simulink subsystem "MultibodySuspensionSSC"  (R2023b)
settings: Solver=VariableStepAuto  StartTime=0.0  StopTime=10.0  RelTol=1e-3
undefined symbols (not defined in the file): EnvGrvty, FrntRef, LAc, LAf, LAr, PlntVehDstCGFrntAxl, PlntVehDstCGRearAxl, PlntVehMass, PlntVehMultiBody, PlntVehMultiBodyGeom, RearRef, StrRodFL, StrRodFR, StrRodRL, StrRodRR, UAc, UAf, UAr, WheelFL, WheelFR, WheelRL, WheelRR, X, Y, Z
libraries: sm_lib x450, fl_lib x96, nesl_utility x64, sdl_lib x8
(part 1 of 18)
settings Model: Creator=The MathWorks, Inc.  LastModifiedBy=The MathWorks, Inc.
settings OptimizationCC: ReuseModelBlockBuffer=off
settings DebuggingCC: SubsystemReferenceDiagnosticForUnitTest=warning

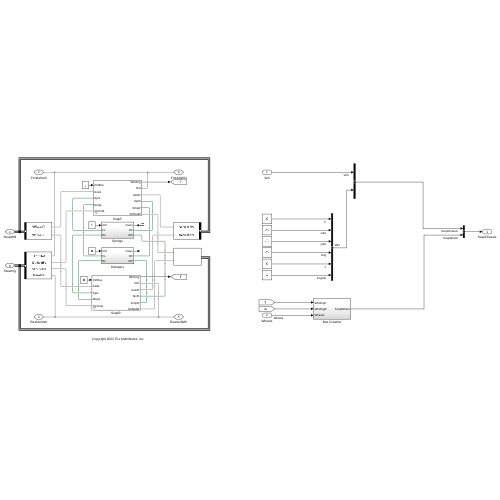
[thumbnail: Simulink's stored preview of the top-level diagram]
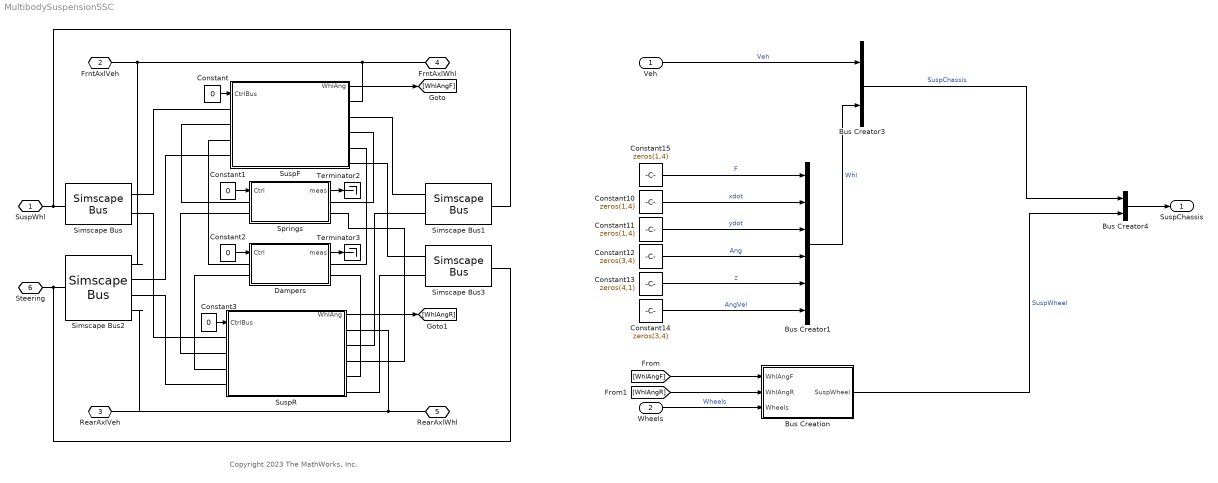
== system MultibodySuspensionSSC ==
  note: Copyright 2023 The MathWorks, Inc.
  Veh : Inport
  Wheels : Inport  Port=2
  Bus Creator1 : BusCreator  Inputs=6
  Bus Creator3 : BusCreator  Inputs=2
  Bus Creator4 : BusCreator  Inputs=2
  Bus Creation : Subsystem
  Constant{,1..3} (4 alike) : Constant  Value=0  SampleTime=-1
  Constant10 : Constant  Value=zeros(1,4)  SampleTime=-1
  Constant11 : Constant  Value=zeros(1,4)  SampleTime=-1
  Constant12 : Constant  Value=zeros(3,4)  SampleTime=-1
  Constant13 : Constant  Value=zeros(4,1)  SampleTime=-1
  Constant14 : Constant  Value=zeros(3,4)  SampleTime=-1
  Constant15 : Constant  Value=zeros(1,4)  SampleTime=-1
  Dampers : Subsystem
  Simscape Bus : SimscapeBus  HierarchyStrings=WheelFL;WheelRL
  Simscape Bus1 : SimscapeBus  HierarchyStrings=WheelFR;WheelRR
  Simscape Bus2 : SimscapeBus  HierarchyStrings=FrntRef;StrRodFL;StrRodRL;RearRef
  Simscape Bus3 : SimscapeBus  HierarchyStrings=StrRodFR;StrRodRR
  Springs : Subsystem
  SuspF : Subsystem  mask(Suspension and Steering){Susp=PlntVehMultiBody.Chassis.SuspF, Init=[0 0 0], InitTriggerDropdown=1}
      mask prompts: Susp "Suspension Parameters"; Init "Initial Values"; InitTriggerDropdown "Initialization Trigger Dropdown"
      mask help: Suspension and steering system for front or rear axle.
      mask init:
      | % curblk = gcb;
      | % Trigger Mask Initialization for 
      | % variant subsystems below this level
      | % sm_car_4post_lib_maskInitTrigger(curblk)
      settings: LibrarySourceBlock=sm_car_4post_lib/Suspension and Steering
      mask TypeOptions InitTriggerDropdown: 0 | 1
  SuspR : Subsystem  mask(Suspension and Steering){Susp=PlntVehMultiBody.Chassis.SuspR, Init=[0 0 0], InitTriggerDropdown=1}
      mask prompts: Susp "Suspension Parameters"; Init "Initial Values"; InitTriggerDropdown "Initialization Trigger Dropdown"
      mask help: Suspension and steering system for front or rear axle.
      mask init:
      | % curblk = gcb;
      | % Trigger Mask Initialization for 
      | % variant subsystems below this level
      | % sm_car_4post_lib_maskInitTrigger(curblk)
      settings: LibrarySourceBlock=sm_car_4post_lib/Suspension and Steering
      mask TypeOptions InitTriggerDropdown: 0 | 1
  Terminator2 : Terminator
  Terminator3 : Terminator
  SuspWhl : PMIOPort  Side=Right
  FrntAxlVeh : PMIOPort  Port=2  Side=Left
  RearAxlVeh : PMIOPort  Port=3  Side=Left
  FrntAxlWhl : PMIOPort  Port=4  Side=Right
  RearAxlWhl : PMIOPort  Port=5  Side=Right
  Steering : PMIOPort  Port=6  Side=Left
  SuspChassis : Outport
  wires:
  Constant10/1 -> Bus Creator1/2  "xdot"
  Veh/1 -> Bus Creator3/1  "Veh"
  Bus Creator3/1 -> Bus Creator4/1  "SuspChassis"
  Bus Creator4/1 -> SuspChassis/1
  Bus Creator1/1 -> Bus Creator3/2  "Whl"
  Constant11/1 -> Bus Creator1/3  "ydot"
  Constant12/1 -> Bus Creator1/4  "Ang"
  Constant13/1 -> Bus Creator1/5  "z"
  Constant14/1 -> Bus Creator1/6  "AngVel"
  Constant15/1 -> Bus Creator1/1  "F"
  Springs/1(meas) -> Terminator2/1
  Dampers/1(meas) -> Terminator3/1
  Constant1/1 -> Springs/1(Ctrl)
  Constant2/1 -> Dampers/1(Ctrl)
  Constant3/1 -> SuspR/1(CtrlBus)
  Constant/1 -> SuspF/1(CtrlBus)
  SuspF/1(WhlAng) -> [WhlAngF]
  SuspR/1(WhlAng) -> [WhlAngR]
  [WhlAngF] -> Bus Creation/1(WhlAngF)
  [WhlAngR] -> Bus Creation/2(WhlAngR)
  Wheels/1 -> Bus Creation/3(Wheels)  "Wheels"
  Bus Creation/1(SuspWheel) -> Bus Creator4/2  "SuspWheel"
  connections:
  Simscape Bus2/RConn1 -- Simscape Bus3/RConn1 -- Steering/RConn1
  SuspF/RConn1 -- FrntAxlVeh/RConn1 -- Simscape Bus2/LConn1 -- FrntAxlWhl/RConn1
  SuspR/RConn1 -- RearAxlWhl/RConn1 -- RearAxlVeh/RConn1 -- Simscape Bus2/LConn4
  SuspWhl/RConn1 -- Simscape Bus1/RConn1 -- Simscape Bus/RConn1
  SuspR/LConn4 -- Simscape Bus2/LConn3
  SuspR/RConn5 -- Simscape Bus3/LConn2
  SuspF/RConn5 -- Simscape Bus3/LConn1
  SuspF/LConn4 -- Simscape Bus2/LConn2
  Springs/LConn2 -- SuspR/LConn2
  Springs/RConn2 -- SuspR/RConn3
  SuspR/RConn4 -- Dampers/RConn2
  SuspR/LConn3 -- Dampers/LConn2
  SuspF/LConn2 -- Springs/LConn1
  SuspF/RConn3 -- Springs/RConn1
  SuspF/LConn3 -- Dampers/LConn1
  SuspF/RConn4 -- Dampers/RConn1
  SuspF/LConn1 -- Simscape Bus/LConn1
  Simscape Bus/LConn2 -- SuspR/LConn1
  SuspF/RConn2 -- Simscape Bus1/LConn1
  Simscape Bus1/LConn2 -- SuspR/RConn2

== system MultibodySuspensionSSC/Bus Creation ==
  WhlAngF : Inport
  WhlAngR : Inport  Port=2
  Wheels : Inport  Port=3
  Bus Creator : BusCreator  Inputs=8
  Bus Selector : BusSelector  OutputSignals=Wheels.Gamma
  Constant{4..9} (6 alike) : Constant  Value=zeros(1,4)  SampleTime=-1
  Convert +Z down : UnaryMinus
  Convert +Z down1 : UnaryMinus
  Matrix Concatenate : Concatenate  Mode=Multidimensional array
  Matrix Concatenate1 : Concatenate  Mode=Multidimensional array  ConcatenateDimension=2
  Reshape : Reshape  OutputDimensionality=Row vector (2-D)
  SuspWheel : Outport
  wires:
  Constant5/1 -> Bus Creator/3  "Vx"
  Wheels/1 -> Bus Selector/1, Bus Creator/8
  Bus Selector/1 -> Reshape/1  "<Gamma>"
  Constant4/1 -> Bus Creator/2  "YawRate"
  Constant8/1 -> Bus Creator/6  "Fext"
  Reshape/1 -> Matrix Concatenate/1
  Matrix Concatenate/1 -> Bus Creator/1  "WhlAng"
  Constant6/1 -> Bus Creator/4  "Vy"
  WhlAngF/1 -> Convert +Z down/1
  Constant9/1 -> Bus Creator/7  "dz"
  Constant7/1 -> Bus Creator/5  "Vz"
  Matrix Concatenate1/1 -> Matrix Concatenate/2
  Convert +Z down/1 -> Matrix Concatenate1/1
  Convert +Z down1/1 -> Matrix Concatenate1/2
  Bus Creator/1 -> SuspWheel/1  "SuspWheel"
  WhlAngR/1 -> Convert +Z down1/1

== system MultibodySuspensionSSC/Dampers ==
  Ctrl : Inport
  Independent : Subsystem  VariantControl=Independent
  Terminator : Terminator
  FL : PMIOPort  Side=Left
  FR : PMIOPort  Port=2  Side=Right
  RL : PMIOPort  Port=3  Side=Left
  RR : PMIOPort  Port=4  Side=Right
  meas : Outport  VectorParamsAs1DForOutWhenUnconnected=off
  wires:
  Ctrl/1 -> Terminator/1
  Independent/1(meas) -> meas/1
  connections:
  Independent/RConn2 -- RR/RConn1
  Independent/RConn1 -- FR/RConn1
  Independent/LConn2 -- RL/RConn1
  Independent/LConn1 -- FL/RConn1

== system MultibodySuspensionSSC/Springs ==
  Ctrl : Inport
  Independent : Subsystem  VariantControl=Independent
  Terminator : Terminator
  FL : PMIOPort  Side=Left
  FR : PMIOPort  Port=2  Side=Right
  RL : PMIOPort  Port=3  Side=Left
  RR : PMIOPort  Port=4  Side=Right
  meas : Outport  VectorParamsAs1DForOutWhenUnconnected=off
  wires:
  Ctrl/1 -> Terminator/1
  Independent/1(meas) -> meas/1
  connections:
  Independent/RConn2 -- RR/RConn1
  Independent/RConn1 -- FR/RConn1
  Independent/LConn1 -- FL/RConn1
  Independent/LConn2 -- RL/RConn1

== system MultibodySuspensionSSC/SuspF ==
  CtrlBus : Inport
  Linkage : Subsystem  VariantControl=Linkage
  Terminator : Terminator
  AxleL : PMIOPort  Side=Left
  Ref : PMIOPort  Port=2  Side=Right
  AxleR : PMIOPort  Port=3  Side=Right
  SprL : PMIOPort  Port=4  Side=Left
  SprR : PMIOPort  Port=5  Side=Right
  DmpL : PMIOPort  Port=6  Side=Left
  DmpR : PMIOPort  Port=7  Side=Right
  StrRodL : PMIOPort  Port=8  Side=Left
  StrRodR : PMIOPort  Port=9  Side=Right
  WhlAng : Outport
  wires:
  CtrlBus/1 -> Terminator/1
  Linkage/1(WhlAng) -> WhlAng/1
  connections:
  Linkage/RConn5 -- StrRodR/RConn1
  StrRodL/RConn1 -- Linkage/LConn4
  Linkage/LConn3 -- DmpL/RConn1
  Linkage/RConn2 -- AxleR/RConn1
  Linkage/LConn2 -- SprL/RConn1
  Linkage/RConn4 -- DmpR/RConn1
  Linkage/RConn3 -- SprR/RConn1
  Linkage/RConn1 -- Ref/RConn1
  Linkage/LConn1 -- AxleL/RConn1

== system MultibodySuspensionSSC/SuspR ==
  CtrlBus : Inport
  Linkage : Subsystem  VariantControl=Linkage
  Terminator : Terminator
  AxleL : PMIOPort  Side=Left
  Ref : PMIOPort  Port=2  Side=Right
  AxleR : PMIOPort  Port=3  Side=Right
  SprL : PMIOPort  Port=4  Side=Left
  SprR : PMIOPort  Port=5  Side=Right
  DmpL : PMIOPort  Port=6  Side=Left
  DmpR : PMIOPort  Port=7  Side=Right
  StrRodL : PMIOPort  Port=8  Side=Left
  StrRodR : PMIOPort  Port=9  Side=Right
  WhlAng : Outport
  wires:
  CtrlBus/1 -> Terminator/1
  Linkage/1(WhlAng) -> WhlAng/1
  connections:
  Linkage/RConn5 -- StrRodR/RConn1
  StrRodL/RConn1 -- Linkage/LConn4
  Linkage/LConn1 -- AxleL/RConn1
  Linkage/RConn1 -- Ref/RConn1
  Linkage/RConn3 -- SprR/RConn1
  Linkage/RConn4 -- DmpR/RConn1
  Linkage/LConn2 -- SprL/RConn1
  Linkage/RConn2 -- AxleR/RConn1
  Linkage/LConn3 -- DmpL/RConn1

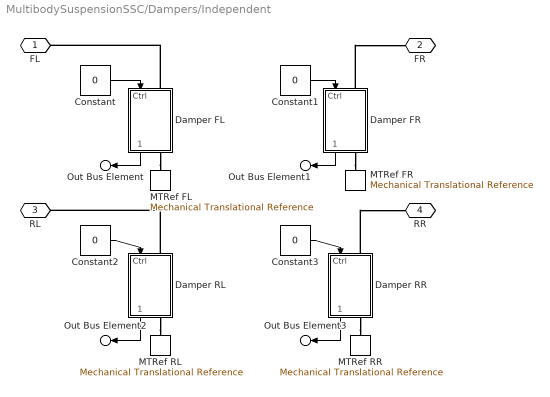
== system MultibodySuspensionSSC/Dampers/Independent ==
  Constant{,1..3} (4 alike) : Constant  Value=0  SampleTime=-1
  Damper FL : Subsystem  mask(Damper){Damper=PlntVehMultiBody.Chassis.Damper.Front}
      mask prompts: Damper "Damper Parameters"
      settings: LibrarySourceBlock=sm_car_4post_lib/Damper
  Damper FR : Subsystem  mask(Damper){Damper=PlntVehMultiBody.Chassis.Damper.Front}
      mask prompts: Damper "Damper Parameters"
      settings: LibrarySourceBlock=sm_car_4post_lib/Damper
  Damper RL : Subsystem  mask(Damper){Damper=PlntVehMultiBody.Chassis.Damper.Rear}
      mask prompts: Damper "Damper Parameters"
      settings: LibrarySourceBlock=sm_car_4post_lib/Damper
  Damper RR : Subsystem  mask(Damper){Damper=PlntVehMultiBody.Chassis.Damper.Rear}
      mask prompts: Damper "Damper Parameters"
      settings: LibrarySourceBlock=sm_car_4post_lib/Damper
  MTRef FL : fl_lib/Mechanical/Translational Elements/Mechanical Translational Reference
  MTRef FR : fl_lib/Mechanical/Translational Elements/Mechanical Translational Reference
  MTRef RL : fl_lib/Mechanical/Translational Elements/Mechanical Translational Reference
  MTRef RR : fl_lib/Mechanical/Translational Elements/Mechanical Translational Reference
  FL : PMIOPort  Side=Left
  FR : PMIOPort  Port=2  Side=Right
  RL : PMIOPort  Port=3  Side=Left
  RR : PMIOPort  Port=4  Side=Right
  Out Bus Element : Outport  VectorParamsAs1DForOutWhenUnconnected=off  PortName=meas  Element=FL
  Out Bus Element1 : Outport  VectorParamsAs1DForOutWhenUnconnected=off  PortName=meas  Element=FR
  Out Bus Element2 : Outport  VectorParamsAs1DForOutWhenUnconnected=off  PortName=meas  Element=RL
  Out Bus Element3 : Outport  VectorParamsAs1DForOutWhenUnconnected=off  PortName=meas  Element=RR
  wires:
  Constant3/1 -> Damper RR/1(Ctrl)
  Constant2/1 -> Damper RL/1(Ctrl)
  Constant1/1 -> Damper FR/1(Ctrl)
  Constant/1 -> Damper FL/1(Ctrl)
  Damper RR/1(meas) -> Out Bus Element3/1
  Damper RL/1(meas) -> Out Bus Element2/1
  Damper FR/1(meas) -> Out Bus Element1/1
  Damper FL/1(meas) -> Out Bus Element/1
  connections:
  Damper FL/RConn1 -- MTRef FL/LConn1
  Damper FL/LConn1 -- FL/RConn1
  Damper RL/RConn1 -- MTRef RL/LConn1
  Damper RL/LConn1 -- RL/RConn1
  Damper RR/RConn1 -- MTRef RR/LConn1
  Damper RR/LConn1 -- RR/RConn1
  Damper FR/RConn1 -- MTRef FR/LConn1
  Damper FR/LConn1 -- FR/RConn1

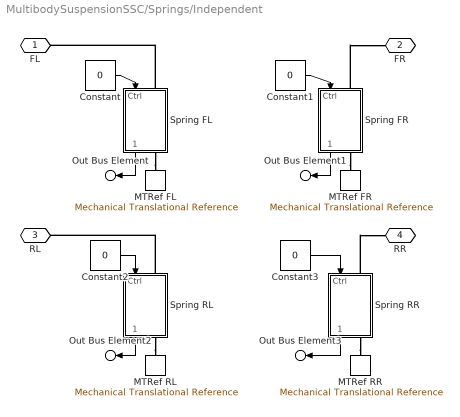
== system MultibodySuspensionSSC/Springs/Independent ==
  Constant{,1..3} (4 alike) : Constant  Value=0  SampleTime=-1
  MTRef FL : fl_lib/Mechanical/Translational Elements/Mechanical Translational Reference
  MTRef FR : fl_lib/Mechanical/Translational Elements/Mechanical Translational Reference
  MTRef RL : fl_lib/Mechanical/Translational Elements/Mechanical Translational Reference
  MTRef RR : fl_lib/Mechanical/Translational Elements/Mechanical Translational Reference
  Spring FL : Subsystem  mask(Spring){Spring=PlntVehMultiBody.Chassis.Spring.Front}
      mask prompts: Spring "Spring Parameters"
      settings: LibrarySourceBlock=sm_car_4post_lib/Spring
  Spring FR : Subsystem  mask(Spring){Spring=PlntVehMultiBody.Chassis.Spring.Front}
      mask prompts: Spring "Spring Parameters"
      settings: LibrarySourceBlock=sm_car_4post_lib/Spring
  Spring RL : Subsystem  mask(Spring){Spring=PlntVehMultiBody.Chassis.Spring.Rear}
      mask prompts: Spring "Spring Parameters"
      settings: LibrarySourceBlock=sm_car_4post_lib/Spring
  Spring RR : Subsystem  mask(Spring){Spring=PlntVehMultiBody.Chassis.Spring.Rear}
      mask prompts: Spring "Spring Parameters"
      settings: LibrarySourceBlock=sm_car_4post_lib/Spring
  FL : PMIOPort  Side=Left
  FR : PMIOPort  Port=2  Side=Right
  RL : PMIOPort  Port=3  Side=Left
  RR : PMIOPort  Port=4  Side=Right
  Out Bus Element : Outport  VectorParamsAs1DForOutWhenUnconnected=off  PortName=meas  Element=FL
  Out Bus Element1 : Outport  VectorParamsAs1DForOutWhenUnconnected=off  PortName=meas  Element=FR
  Out Bus Element2 : Outport  VectorParamsAs1DForOutWhenUnconnected=off  PortName=meas  Element=RL
  Out Bus Element3 : Outport  VectorParamsAs1DForOutWhenUnconnected=off  PortName=meas  Element=RR
  wires:
  Constant3/1 -> Spring RR/1(Ctrl)
  Constant2/1 -> Spring RL/1(Ctrl)
  Constant1/1 -> Spring FR/1(Ctrl)
  Constant/1 -> Spring FL/1(Ctrl)
  Spring RR/1(meas) -> Out Bus Element3/1
  Spring RL/1(meas) -> Out Bus Element2/1
  Spring FR/1(meas) -> Out Bus Element1/1
  Spring FL/1(meas) -> Out Bus Element/1
  connections:
  Spring FL/RConn1 -- MTRef FL/LConn1
  Spring FL/LConn1 -- FL/RConn1
  Spring RL/RConn1 -- MTRef RL/LConn1
  Spring RL/LConn1 -- RL/RConn1
  Spring RR/RConn1 -- MTRef RR/LConn1
  Spring RR/LConn1 -- RR/RConn1
  Spring FR/RConn1 -- MTRef FR/LConn1
  Spring FR/LConn1 -- FR/RConn1

== system MultibodySuspensionSSC/SuspF/Linkage ==
  Anti Roll Bar : Subsystem  Variant=on  VariantControlMode=label  LabelModeActiveChoice=Simple  mask{AntiRollBar=Susp.AntiRollBar, VariantLabel=Susp.AntiRollBar.class.Value, InitTriggerDropdown=1}
      mask prompts: AntiRollBar "Anti-Roll Bar"; VariantLabel "Variant Label"; InitTriggerDropdown "Initialization Trigger Dropdown"
      settings: AttributesFormatString=%<LabelModeActiveChoice>
      mask TypeOptions InitTriggerDropdown: 0 | 1
  Linkage L : Subsystem  Variant=on  VariantControlMode=label  VariantControl=Variant1  LabelModeActiveChoice=DoubleWishbone  mask(Suspension){popup_leftRight=Left, Linkage=Susp.Linkage, Init=[0 0 0], VariantLabel=Susp.Linkage.class.Value, InitTriggerDropdown=1}
      mask prompts: popup_leftRight "Left/Right"; Linkage "Linkage Parameters"; Init "Initial Values"; VariantLabel "Variant Label"; InitTriggerDropdown "Initialization Trigger Dropdown"
      mask help: Suspension with multiple variants. Variants are configured by parameter Variant Label. Parameter values are contained within Linkage Parameters.
      mask init:
      | % curblk = gcb;
      | 
      | % Set variant for this block 
      | % set_param(curblk,'LabelModeActiveChoice',VariantLabel);
      | 
      | % Trigger Mask Initialization for 
      | % variant subsystems below this level
      | % sm_car_4post_lib_maskInitTrigger(curblk)
      | 
      | % Set Left/Right fields
      | 
      | % sm_car_4post_lib_setLeftRight(curblk,'variant');
      settings: AttributesFormatString=%<ActiveVariant>  LibrarySourceBlock=sm_car_4post_lib/Suspension and Steering/Linkage/Linkage L
      mask TypeOptions popup_leftRight: Left | Right
      mask TypeOptions InitTriggerDropdown: 0 | 1
  Linkage R : Subsystem  Variant=on  VariantControlMode=label  VariantControl=Variant1  LabelModeActiveChoice=DoubleWishbone  mask(Suspension){popup_leftRight=Right, Linkage=Susp.Linkage, Init=[0 0 0], VariantLabel=Susp.Linkage.class.Value, InitTriggerDropdown=1}
      mask prompts: popup_leftRight "Left/Right"; Linkage "Linkage Parameters"; Init "Initial Values"; VariantLabel "Variant Label"; InitTriggerDropdown "Initialization Trigger Dropdown"
      mask help: Suspension with multiple variants. Variants are configured by parameter Variant Label. Parameter values are contained within Linkage Parameters.
      mask init:
      | % curblk = gcb;
      | 
      | % % Set variant for this block 
      | % set_param(curblk,'LabelModeActiveChoice',VariantLabel);
      | 
      | % Trigger Mask Initialization for 
      | % variant subsystems below this level
      | % sm_car_4post_lib_maskInitTrigger(curblk)
      | 
      | % Set Left/Right fields
      | 
      | % sm_car_4post_lib_setLeftRight(curblk,'variant');
      settings: AttributesFormatString=%<ActiveVariant>  LibrarySourceBlock=sm_car_4post_lib/Suspension and Steering/Linkage/Linkage R
      mask TypeOptions popup_leftRight: Left | Right
      mask TypeOptions InitTriggerDropdown: 0 | 1
  Matrix Concatenate : Concatenate  Mode=Multidimensional array  ConcatenateDimension=2
  AxleL : PMIOPort  Side=Left
  Ref : PMIOPort  Port=2  Side=Right
  AxleR : PMIOPort  Port=3  Side=Right
  SprL : PMIOPort  Port=4  Side=Left
  SprR : PMIOPort  Port=5  Side=Right
  DmpL : PMIOPort  Port=6  Side=Left
  DmpR : PMIOPort  Port=7  Side=Right
  StrRodL : PMIOPort  Port=8  Side=Left
  StrRodR : PMIOPort  Port=9  Side=Right
  WhlAng : Outport
  wires:
  Matrix Concatenate/1 -> WhlAng/1
  Linkage L/1(WhlAng) -> Matrix Concatenate/1
  Linkage R/1(WhlAng) -> Matrix Concatenate/2
  connections:
  Linkage L/RConn1 -- StrRodL/RConn1
  Linkage L/LConn3 -- DmpL/RConn1
  Linkage L/LConn2 -- SprL/RConn1
  Linkage R/LConn1 -- AxleR/RConn1
  Linkage L/LConn1 -- AxleL/RConn1
  Linkage R/RConn2 -- Ref/RConn1 -- Anti Roll Bar/LConn2 -- Linkage L/RConn2
  Linkage R/RConn1 -- StrRodR/RConn1
  Linkage R/LConn3 -- DmpR/RConn1
  Linkage R/LConn2 -- SprR/RConn1
  Linkage L/LConn4 -- Anti Roll Bar/LConn1
  Linkage R/LConn4 -- Anti Roll Bar/LConn3

== system MultibodySuspensionSSC/SuspR/Linkage ==
  Anti Roll Bar : Subsystem  Variant=on  VariantControlMode=label  LabelModeActiveChoice=Simple  mask{AntiRollBar=Susp.AntiRollBar, VariantLabel=Susp.AntiRollBar.class.Value, InitTriggerDropdown=1}
      mask prompts: AntiRollBar "Anti-Roll Bar"; VariantLabel "Variant Label"; InitTriggerDropdown "Initialization Trigger Dropdown"
      settings: AttributesFormatString=%<LabelModeActiveChoice>
      mask TypeOptions InitTriggerDropdown: 0 | 1
  Linkage L : Subsystem  Variant=on  VariantControlMode=label  VariantControl=Variant1  LabelModeActiveChoice=DoubleWishbone  mask(Suspension){popup_leftRight=Left, Linkage=Susp.Linkage, Init=[0 0 0], VariantLabel=Susp.Linkage.class.Value, InitTriggerDropdown=1}
      mask prompts: popup_leftRight "Left/Right"; Linkage "Linkage Parameters"; Init "Initial Values"; VariantLabel "Variant Label"; InitTriggerDropdown "Initialization Trigger Dropdown"
      mask help: Suspension with multiple variants. Variants are configured by parameter Variant Label. Parameter values are contained within Linkage Parameters.
      mask init: same as MultibodySuspensionSSC/SuspF/Linkage/Linkage L
      settings: AttributesFormatString=%<ActiveVariant>  LibrarySourceBlock=sm_car_4post_lib/Suspension and Steering/Linkage/Linkage L
      mask TypeOptions popup_leftRight: Left | Right
      mask TypeOptions InitTriggerDropdown: 0 | 1
  Linkage R : Subsystem  Variant=on  VariantControlMode=label  VariantControl=Variant1  LabelModeActiveChoice=DoubleWishbone  mask(Suspension){popup_leftRight=Right, Linkage=Susp.Linkage, Init=[0 0 0], VariantLabel=Susp.Linkage.class.Value, InitTriggerDropdown=1}
      mask prompts: popup_leftRight "Left/Right"; Linkage "Linkage Parameters"; Init "Initial Values"; VariantLabel "Variant Label"; InitTriggerDropdown "Initialization Trigger Dropdown"
      mask help: Suspension with multiple variants. Variants are configured by parameter Variant Label. Parameter values are contained within Linkage Parameters.
      mask init: same as MultibodySuspensionSSC/SuspF/Linkage/Linkage R
      settings: AttributesFormatString=%<ActiveVariant>  LibrarySourceBlock=sm_car_4post_lib/Suspension and Steering/Linkage/Linkage R
      mask TypeOptions popup_leftRight: Left | Right
      mask TypeOptions InitTriggerDropdown: 0 | 1
  Matrix Concatenate : Concatenate  Mode=Multidimensional array  ConcatenateDimension=2
  AxleL : PMIOPort  Side=Left
  Ref : PMIOPort  Port=2  Side=Right
  AxleR : PMIOPort  Port=3  Side=Right
  SprL : PMIOPort  Port=4  Side=Left
  SprR : PMIOPort  Port=5  Side=Right
  DmpL : PMIOPort  Port=6  Side=Left
  DmpR : PMIOPort  Port=7  Side=Right
  StrRodL : PMIOPort  Port=8  Side=Left
  StrRodR : PMIOPort  Port=9  Side=Right
  WhlAng : Outport
  wires:
  Matrix Concatenate/1 -> WhlAng/1
  Linkage L/1(WhlAng) -> Matrix Concatenate/1
  Linkage R/1(WhlAng) -> Matrix Concatenate/2
  connections:
  Linkage R/LConn2 -- SprR/RConn1
  Linkage R/LConn3 -- DmpR/RConn1
  Linkage R/RConn1 -- StrRodR/RConn1
  Linkage R/RConn2 -- Anti Roll Bar/LConn2 -- Ref/RConn1 -- Linkage L/RConn2
  Linkage L/LConn1 -- AxleL/RConn1
  Linkage R/LConn1 -- AxleR/RConn1
  Linkage L/LConn2 -- SprL/RConn1
  Linkage L/LConn3 -- DmpL/RConn1
  Linkage L/RConn1 -- StrRodL/RConn1
  Anti Roll Bar/LConn1 -- Linkage L/LConn4
  Anti Roll Bar/LConn3 -- Linkage R/LConn4

== system MultibodySuspensionSSC/Dampers/Independent/Damper FL ==
  Ctrl : Inport
  Damper : Subsystem  Variant=on  VariantControlMode=label  VariantControl=Linear  LabelModeActiveChoice=Linear
  R : PMIOPort  Side=Left
  C : PMIOPort  Port=2  Side=Right
  meas : Outport  VectorParamsAs1DForOutWhenUnconnected=off
  wires:
  Damper/1(meas) -> meas/1
  Ctrl/1 -> Damper/1(Ctrl)
  connections:
  Damper/RConn1 -- C/RConn1
  Damper/LConn1 -- R/RConn1

== system MultibodySuspensionSSC/Dampers/Independent/Damper FR ==
  Ctrl : Inport
  Damper : Subsystem  Variant=on  VariantControlMode=label  VariantControl=Linear  LabelModeActiveChoice=Linear
  R : PMIOPort  Side=Left
  C : PMIOPort  Port=2  Side=Right
  meas : Outport  VectorParamsAs1DForOutWhenUnconnected=off
  wires:
  Damper/1(meas) -> meas/1
  Ctrl/1 -> Damper/1(Ctrl)
  connections:
  Damper/LConn1 -- R/RConn1
  Damper/RConn1 -- C/RConn1

== system MultibodySuspensionSSC/Dampers/Independent/Damper RL ==
  Ctrl : Inport
  Damper : Subsystem  Variant=on  VariantControlMode=label  VariantControl=Linear  LabelModeActiveChoice=Linear
  R : PMIOPort  Side=Left
  C : PMIOPort  Port=2  Side=Right
  meas : Outport  VectorParamsAs1DForOutWhenUnconnected=off
  wires:
  Damper/1(meas) -> meas/1
  Ctrl/1 -> Damper/1(Ctrl)
  connections:
  Damper/LConn1 -- R/RConn1
  Damper/RConn1 -- C/RConn1

== system MultibodySuspensionSSC/Dampers/Independent/Damper RR ==
  Ctrl : Inport
  Damper : Subsystem  Variant=on  VariantControlMode=label  VariantControl=Linear  LabelModeActiveChoice=Linear
  R : PMIOPort  Side=Left
  C : PMIOPort  Port=2  Side=Right
  meas : Outport  VectorParamsAs1DForOutWhenUnconnected=off
  wires:
  Damper/1(meas) -> meas/1
  Ctrl/1 -> Damper/1(Ctrl)
  connections:
  Damper/LConn1 -- R/RConn1
  Damper/RConn1 -- C/RConn1

== system MultibodySuspensionSSC/Springs/Independent/Spring FL ==
  Ctrl : Inport
  Spring : Subsystem  Variant=on  VariantControlMode=label  VariantControl=Linear  LabelModeActiveChoice=Linear
  R : PMIOPort  Side=Left
  C : PMIOPort  Port=2  Side=Right
  meas : Outport  VectorParamsAs1DForOutWhenUnconnected=off
  wires:
  Spring/1(meas) -> meas/1
  Ctrl/1 -> Spring/1(Ctrl)
  connections:
  Spring/RConn1 -- C/RConn1
  Spring/LConn1 -- R/RConn1

== system MultibodySuspensionSSC/Springs/Independent/Spring FR ==
  Ctrl : Inport
  Spring : Subsystem  Variant=on  VariantControlMode=label  VariantControl=Linear  LabelModeActiveChoice=Linear
  R : PMIOPort  Side=Left
  C : PMIOPort  Port=2  Side=Right
  meas : Outport  VectorParamsAs1DForOutWhenUnconnected=off
  wires:
  Ctrl/1 -> Spring/1(Ctrl)
  Spring/1(meas) -> meas/1
  connections:
  Spring/RConn1 -- C/RConn1
  Spring/LConn1 -- R/RConn1

== system MultibodySuspensionSSC/Springs/Independent/Spring RL ==
  Ctrl : Inport
  Spring : Subsystem  Variant=on  VariantControlMode=label  VariantControl=Linear  LabelModeActiveChoice=Linear
  R : PMIOPort  Side=Left
  C : PMIOPort  Port=2  Side=Right
  meas : Outport  VectorParamsAs1DForOutWhenUnconnected=off
  wires:
  Ctrl/1 -> Spring/1(Ctrl)
  Spring/1(meas) -> meas/1
  connections:
  Spring/RConn1 -- C/RConn1
  Spring/LConn1 -- R/RConn1

== system MultibodySuspensionSSC/Springs/Independent/Spring RR ==
  Ctrl : Inport
  Spring : Subsystem  Variant=on  VariantControlMode=label  VariantControl=Linear  LabelModeActiveChoice=Linear
  R : PMIOPort  Side=Left
  C : PMIOPort  Port=2  Side=Right
  meas : Outport  VectorParamsAs1DForOutWhenUnconnected=off
  wires:
  Ctrl/1 -> Spring/1(Ctrl)
  Spring/1(meas) -> meas/1
  connections:
  Spring/RConn1 -- C/RConn1
  Spring/LConn1 -- R/RConn1

== system MultibodySuspensionSSC/SuspF/Linkage/Anti Roll Bar ==
  " None" : Subsystem  VariantControl=None  mask(Anti-Roll Bar Placeholder){}
      mask help: Empty subsystem, used as a variant that omits an anti-roll bar.
  Simple : Subsystem  VariantControl=Simple  mask(Anti-Roll Bar, Simple){k=AntiRollBar.k.Value}
      mask prompts: k "Stiffness"
      mask help: Models an anti-roll bar by applying un-opposed forces to suspension arms. Conceptual use only.
  LAoL : PMIOPort  Side=Left
  Ref : PMIOPort  Port=2  Side=Left
  LAoR : PMIOPort  Port=3  Side=Left

== system MultibodySuspensionSSC/SuspF/Linkage/Linkage L ==
  DoubleWishbone : Subsystem  VariantControl=DoubleWishbone  mask(Double-Wishbone Suspension){popup_leftRight=Left, hp_in_f_ua=Linkage.UpperWishbone.sInboardF.Value, hp_in_r_ua=Linkage.UpperWishbone.sInboardR.Value, hp_out_ua=Linkage.UpperWishbone.sOutboard.Value, hp_in_f_la=Linkage.LowerWishbone.sInboardF.Value, hp_in_r_la=Linkage.LowerWishbone.sInboardR.Value, hp_out_la=Linkage.LowerWishbone.sOutboard.Value, hp_upr_cg=Linkage.Upright.sCG.Value, hp_upr_wc=Linkage.Upright.sWheelCentre.Value, hp_in_rod=Linkage.TrackRod.sInboard.Value, hp_upr_rod=Linkage.TrackRod.sOutboard.Value, hp_spr_top=Linkage.Shock.sTop.Value, hp_spr_bot=Linkage.Shock.sBottom.Value, clr_hp=PlntVehMultiBodyGeom.hp.clr, opc_hp=PlntVehMultiBodyGeom.hp.opc, size_hp=0.025, ua_mass=Linkage.UpperWishbone.m.Value, clr_ua=PlntVehMultiBodyGeom.yellow, opc_ua=PlntVehMultiBodyGeom.part.opc, radius_ua=0.02, la_mass=Linkage.LowerWishbone.m.Value, clr_la=PlntVehMultiBodyGeom.yellow, opc_la=PlntVehMultiBodyGeom.part.opc, radius_la=0.02, shock_pist_mass=Linkage.Shock.mPiston.Value, shock_cyl_mass=Linkage.Shock.mCylinder.Value, up_lim_bumpstop=Linkage.Endstop.xMax.Value, low_lim_bumpstop=Linkage.Endstop.xMin.Value, clr_conn_shock=PlntVehMultiBodyGeom.hp.clr, opc_conn_shock=PlntVehMultiBodyGeom.hp.opc, size_conn_shock=0.025, clr_shock_cyl=PlntVehMultiBodyGeom.blue, opc_shock_cyl=1.0, radius_shock_cyl=0.05, clr_shock_piston=PlntVehMultiBodyGeom.gray, opc_shock_piston=1.0, clr_shock_bumpstop=PlntVehMultiBodyGeom.yellowpale, opc_shock_bumpstop=1.0, deadvol_len_shock_cyl=PlntVehMultiBodyGeom.shock.dead_length, piston_len_shock=PlntVehMultiBodyGeom.shock.piston, cyl_cap_len_shock=PlntVehMultiBodyGeom.shock.cap, bumpstop_len_shock=PlntVehMultiBodyGeom.shock.bumpstop_len, upr_mass=Linkage.Upright.m.Value, atoe=Linkage.Upright.aToe.Value, acamber=Linkage.Upright.aCamber.Value, clr_conn_upr=PlntVehMultiBodyGeom.hp.clr, opc_conn_upr=PlntVehMultiBodyGeom.hp.opc, size_conn_upr=PlntVehMultiBodyGeom.hp.rad, clr_upr=PlntVehMultiBodyGeom.green, opc_upr=PlntVehMultiBodyGeom.part.opc, radius_upr=0.02, clr_stub_axle=PlntVehMultiBodyGeom.black, opc_stub_axle=PlntVehMultiBodyGeom.part.opc, radius_stub_axle=0.02, rod_mass=Linkage.TrackRod.m.Value, clr_conn_rod=PlntVehMultiBodyGeom.hp.clr, opc_conn_rod=PlntVehMultiBodyGeom.hp.opc, size_conn_rod=PlntVehMultiBodyGeom.hp.rad, clr_rod=PlntVehMultiBodyGeom.purple, opc_rod=PlntVehMultiBodyGeom.part.opc, radius_rod=0.02, whl_init_spd_lr=[0 0 0], whlind=1}
      mask prompts: popup_leftRight "Left/Right"; hp_in_f_ua "Upper Arm Front [xyz] (m)"; hp_in_r_ua "Upper Arm Rear [xyz] (m)"; hp_out_ua "Upper Arm Outboard [xyz] (m)"; hp_in_f_la "Lower Arm Front [xyz] (m)"; hp_in_r_la "Lower Arm Rear [xyz] (m)"; hp_out_la "Lower Arm Outboard [xyz] (m)"; hp_upr_cg "Upright CG [xyz] (m)"; hp_upr_wc "Wheel Center [xyz] (m)"; hp_in_rod "Track Rod Inboard [xyz] (m)"; hp_upr_rod "Track Rod Outboard [xyz] (m)"; hp_spr_top "Spring Top [xyz] (m)"; hp_spr_bot "Spring Bottom [xyz] (m)"; ua_mass "Mass (kg)"; clr_ua "Color [RGB]"; opc_ua "Opacity (0-1)"; radius_ua "Radius (m)"; la_mass "Mass (kg)"; clr_la "Color [RGB]"; opc_la "Opacity (0-1)"; radius_la "Radius (m)"; shock_pist_mass "Piston Mass (kg)"; shock_cyl_mass "Cylinder Mass (kg)"; up_lim_bumpstop "Upper Limit (m)"; low_lim_bumpstop "Lower Limit (m)"; deadvol_len_shock_cyl "Dead Volume Height (m)"; piston_len_shock "Piston Length (m)"; cyl_cap_len_shock "Cylinder Cap Length (m)"; bumpstop_len_shock "Bumpstop Length (m)"; upr_mass "Mass (kg)"; atoe "Toe Angle (deg)"; acamber "Camber Angle (deg)"; rod_mass "Mass (kg)"; whl_init_spd_lr "Initial Wheel Speed (rad/s)"; whlind "Wheel Index"
      mask help: This models a double-wishbone suspension for steered and non-steered configurations. The non-steered configuration maintains its orientation via the track rods that connect to fixed points on the subframe.
      mask init:
      | % sm_car_4post_lib_setLeftRight(gcb,'none');
      | 
      | if(popup_leftRight == 1)
      |     rhs_susp = 1;
      |     whlind = 1;
      | elseif(popup_leftRight == 2)
      |     rhs_susp = -1;
      |     whlind = 2;
      | end
      mask TypeOptions popup_leftRight: Left | Right
      mask TypeOptions hp_in_f_ua: Upper Arm/hp_in_f | Hardpoints/hp_in_f_ua
      mask TypeOptions hp_in_r_ua: Upper Arm/hp_in_r | Hardpoints/hp_in_r_ua
      mask TypeOptions hp_out_ua: Upper Arm/hp_out | Upright/hp_ua_out
      mask TypeOptions hp_in_f_la: Lower Arm/hp_in_f | Hardpoints/hp_in_f_la
      mask TypeOptions hp_in_r_la: Lower Arm/hp_in_r | Hardpoints/hp_in_r_la
      mask TypeOptions hp_out_la: Lower Arm/hp_out | Upright/hp_la_out
      mask TypeOptions hp_upr_cg: Upright/hp_upr_cg
      mask TypeOptions hp_upr_wc: Upright/hp_upr_wc
      mask TypeOptions hp_in_rod: Track Rod/hp_in
      mask TypeOptions hp_upr_rod: Track Rod/hp_out | Upright/hp_upr_rod
      mask TypeOptions hp_spr_top: Hardpoints/hp_spr_top | Shock/hp_spr_top
      mask TypeOptions hp_spr_bot: Lower Arm/hp_spr | Shock/hp_spr_bot
      mask TypeOptions clr_hp: Hardpoints/clr_hp
      mask TypeOptions opc_hp: Hardpoints/opc_hp
      mask TypeOptions size_hp: Hardpoints/size_hp
      mask TypeOptions ua_mass: Upper Arm/ua_mass
      mask TypeOptions clr_ua: Upper Arm/clr_ua
      mask TypeOptions opc_ua: Upper Arm/opc_ua
      mask TypeOptions radius_ua: Upper Arm/radius_ua
      mask TypeOptions la_mass: Lower Arm/la_mass
      mask TypeOptions clr_la: Lower Arm/clr_la
      mask TypeOptions opc_la: Lower Arm/opc_la
      mask TypeOptions radius_la: Lower Arm/radius_la
      mask TypeOptions shock_pist_mass: Shock/shock_pist_mass
      mask TypeOptions shock_cyl_mass: Shock/shock_cyl_mass
      mask TypeOptions up_lim_bumpstop: Shock/up_lim_bumpstop
      mask TypeOptions low_lim_bumpstop: Shock/low_lim_bumpstop
      mask TypeOptions clr_conn_shock: Shock/clr_conn_shock
      mask TypeOptions opc_conn_shock: Shock/opc_conn_shock
      mask TypeOptions size_conn_shock: Shock/size_conn_shock
      mask TypeOptions clr_shock_cyl: Shock/clr_shock_cyl
      mask TypeOptions opc_shock_cyl: Shock/opc_shock_cyl
      mask TypeOptions radius_shock_cyl: Shock/radius_shock_cyl
      mask TypeOptions clr_shock_piston: Shock/clr_shock_piston
      mask TypeOptions opc_shock_piston: Shock/opc_shock_piston
      mask TypeOptions clr_shock_bumpstop: Shock/clr_shock_bumpstop
      mask TypeOptions opc_shock_bumpstop: Shock/opc_shock_bumpstop
      mask TypeOptions deadvol_len_shock_cyl: Shock/deadvol_len_shock_cyl
      mask TypeOptions piston_len_shock: Shock/piston_len_shock
      mask TypeOptions cyl_cap_len_shock: Shock/cyl_cap_len_shock
      mask TypeOptions bumpstop_len_shock: Shock/bumpstop_len_shock
      mask TypeOptions upr_mass: Upright/upr_mass
      mask TypeOptions atoe: Upright/atoe
      mask TypeOptions acamber: Upright/acamber
      mask TypeOptions clr_conn_upr: Upright/clr_conn_upr
      mask TypeOptions opc_conn_upr: Upright/opc_conn_upr
      mask TypeOptions size_conn_upr: Upright/size_conn_upr
      mask TypeOptions clr_upr: Upright/clr_upr
      mask TypeOptions opc_upr: Upright/opc_upr
      mask TypeOptions radius_upr: Upright/radius_upr
      mask TypeOptions clr_stub_axle: Upright/clr_stub_axle
      mask TypeOptions opc_stub_axle: Upright/opc_stub_axle
      mask TypeOptions radius_stub_axle: Upright/radius_stub_axle
      mask TypeOptions rod_mass: Track Rod/rod_mass
      mask TypeOptions clr_conn_rod: Track Rod/clr_conn_rod
      mask TypeOptions opc_conn_rod: Track Rod/opc_conn_rod
      mask TypeOptions size_conn_rod: Track Rod/size_conn_rod
      mask TypeOptions clr_rod: Track Rod/clr_rod
      mask TypeOptions opc_rod: Track Rod/opc_rod
      mask TypeOptions radius_rod: Track Rod/radius_rod
      mask DialogControl cont_hp Prompt: Hardpoints
      mask DialogControl cont_vis_hp Prompt: Visualization
      mask DialogControl text_clr_hp Prompt: Color [RGB]
      mask DialogControl text_opc_hp Prompt: Opac. (0-1)
      mask DialogControl text_size_hp Prompt: Size (m)
      mask DialogControl text_hp Prompt: Hardpoints
      mask DialogControl cont_ua Prompt: UA
      mask DialogControl cont_vis_ua Prompt: Visualization
      mask DialogControl cont_la Prompt: LA
      mask DialogControl cont_vis_la Prompt: Visualization
      mask DialogControl cont_shock Prompt: Shock
      mask DialogControl cont_parts Prompt: Parts
      mask DialogControl cont_bumpstop Prompt: Bumpstop
      mask DialogControl cont_vis_shock Prompt: Visualization
      mask DialogControl text_clr_shock Prompt: Color  [RGB]
      mask DialogControl text_opc_shock Prompt: Opac. (0-1)
      mask DialogControl text_size_shock Prompt: Size (m)
      mask DialogControl text_conn_shock Prompt: Connections
      mask DialogControl text_shock_shock Prompt: Cylinder
      mask DialogControl text_shock_piston Prompt: Piston
      mask DialogControl text_piston_radius Prompt: <cylinder radius>
      mask DialogControl text_shock_bumpstop Prompt: Bumpstop
      mask DialogControl text_bumpstop_radius Prompt: <cylinder radius>
      mask DialogControl cont_upright Prompt: Upright
      mask DialogControl grp_upright Prompt: Upright
      mask DialogControl cont_vis_upr Prompt: Visualization
      mask DialogControl text_clr_upr Prompt: Color [RGB]
      mask DialogControl text_opc_upr Prompt: Opac. (0-1)
      mask DialogControl text_size_upr Prompt: Size (m)
      mask DialogControl text_conn_upr Prompt: Connections
      mask DialogControl text_upright Prompt: Upright
      mask DialogControl text_stub_axle Prompt: Stub Axle
      mask DialogControl cont_steer Prompt: Steer
      mask DialogControl grp_rod Prompt: Rod
      mask DialogControl cont_vis_rod Prompt: Visualization
      mask DialogControl text_clr_rod Prompt: Color [RGB]
      mask DialogControl text_opc_rod Prompt: Opac. (0-1)
      mask DialogControl text_size_rod Prompt: Size (m)
      mask DialogControl text_conn_rod Prompt: Connections
      mask DialogControl text_rod_rod Prompt: Rod
      mask DialogControl cont_init Prompt: Initial
  Rack : PMIOPort  Side=Right
  Ref : PMIOPort  Port=2  Side=Right
  Axle : PMIOPort  Port=3  Side=Left
  S : PMIOPort  Port=4  Side=Left
  D : PMIOPort  Port=5  Side=Left
  LAo : PMIOPort  Port=6  Side=Left
  WhlAng : Outport

== system MultibodySuspensionSSC/SuspF/Linkage/Linkage R ==
  DoubleWishbone : Subsystem  VariantControl=DoubleWishbone  mask(Double-Wishbone Suspension){popup_leftRight=Right, hp_in_f_ua=Linkage.UpperWishbone.sInboardF.Value, hp_in_r_ua=Linkage.UpperWishbone.sInboardR.Value, hp_out_ua=Linkage.UpperWishbone.sOutboard.Value, hp_in_f_la=Linkage.LowerWishbone.sInboardF.Value, hp_in_r_la=Linkage.LowerWishbone.sInboardR.Value, hp_out_la=Linkage.LowerWishbone.sOutboard.Value, hp_upr_cg=Linkage.Upright.sCG.Value, hp_upr_wc=Linkage.Upright.sWheelCentre.Value, hp_in_rod=Linkage.TrackRod.sInboard.Value, hp_upr_rod=Linkage.TrackRod.sOutboard.Value, hp_spr_top=Linkage.Shock.sTop.Value, hp_spr_bot=Linkage.Shock.sBottom.Value, clr_hp=PlntVehMultiBodyGeom.hp.clr, opc_hp=PlntVehMultiBodyGeom.hp.opc, size_hp=0.025, ua_mass=Linkage.UpperWishbone.m.Value, clr_ua=PlntVehMultiBodyGeom.yellow, opc_ua=PlntVehMultiBodyGeom.part.opc, radius_ua=0.02, la_mass=Linkage.LowerWishbone.m.Value, clr_la=PlntVehMultiBodyGeom.yellow, opc_la=PlntVehMultiBodyGeom.part.opc, radius_la=0.02, shock_pist_mass=Linkage.Shock.mPiston.Value, shock_cyl_mass=Linkage.Shock.mCylinder.Value, up_lim_bumpstop=Linkage.Endstop.xMax.Value, low_lim_bumpstop=Linkage.Endstop.xMin.Value, clr_conn_shock=PlntVehMultiBodyGeom.hp.clr, opc_conn_shock=PlntVehMultiBodyGeom.hp.opc, size_conn_shock=0.025, clr_shock_cyl=PlntVehMultiBodyGeom.blue, opc_shock_cyl=1.0, radius_shock_cyl=0.05, clr_shock_piston=PlntVehMultiBodyGeom.gray, opc_shock_piston=1.0, clr_shock_bumpstop=PlntVehMultiBodyGeom.yellowpale, opc_shock_bumpstop=1.0, deadvol_len_shock_cyl=PlntVehMultiBodyGeom.shock.dead_length, piston_len_shock=PlntVehMultiBodyGeom.shock.piston, cyl_cap_len_shock=PlntVehMultiBodyGeom.shock.cap, bumpstop_len_shock=PlntVehMultiBodyGeom.shock.bumpstop_len, upr_mass=Linkage.Upright.m.Value, atoe=Linkage.Upright.aToe.Value, acamber=Linkage.Upright.aCamber.Value, clr_conn_upr=PlntVehMultiBodyGeom.hp.clr, opc_conn_upr=PlntVehMultiBodyGeom.hp.opc, size_conn_upr=PlntVehMultiBodyGeom.hp.rad, clr_upr=PlntVehMultiBodyGeom.green, opc_upr=PlntVehMultiBodyGeom.part.opc, radius_upr=0.02, clr_stub_axle=PlntVehMultiBodyGeom.black, opc_stub_axle=PlntVehMultiBodyGeom.part.opc, radius_stub_axle=0.02, rod_mass=Linkage.TrackRod.m.Value, clr_conn_rod=PlntVehMultiBodyGeom.hp.clr, opc_conn_rod=PlntVehMultiBodyGeom.hp.opc, size_conn_rod=PlntVehMultiBodyGeom.hp.rad, clr_rod=PlntVehMultiBodyGeom.purple, opc_rod=PlntVehMultiBodyGeom.part.opc, radius_rod=0.02, whl_init_spd_lr=[0 0 0], whlind=1}
      mask prompts: popup_leftRight "Left/Right"; hp_in_f_ua "Upper Arm Front [xyz] (m)"; hp_in_r_ua "Upper Arm Rear [xyz] (m)"; hp_out_ua "Upper Arm Outboard [xyz] (m)"; hp_in_f_la "Lower Arm Front [xyz] (m)"; hp_in_r_la "Lower Arm Rear [xyz] (m)"; hp_out_la "Lower Arm Outboard [xyz] (m)"; hp_upr_cg "Upright CG [xyz] (m)"; hp_upr_wc "Wheel Center [xyz] (m)"; hp_in_rod "Track Rod Inboard [xyz] (m)"; hp_upr_rod "Track Rod Outboard [xyz] (m)"; hp_spr_top "Spring Top [xyz] (m)"; hp_spr_bot "Spring Bottom [xyz] (m)"; ua_mass "Mass (kg)"; clr_ua "Color [RGB]"; opc_ua "Opacity (0-1)"; radius_ua "Radius (m)"; la_mass "Mass (kg)"; clr_la "Color [RGB]"; opc_la "Opacity (0-1)"; radius_la "Radius (m)"; shock_pist_mass "Piston Mass (kg)"; shock_cyl_mass "Cylinder Mass (kg)"; up_lim_bumpstop "Upper Limit (m)"; low_lim_bumpstop "Lower Limit (m)"; deadvol_len_shock_cyl "Dead Volume Height (m)"; piston_len_shock "Piston Length (m)"; cyl_cap_len_shock "Cylinder Cap Length (m)"; bumpstop_len_shock "Bumpstop Length (m)"; upr_mass "Mass (kg)"; atoe "Toe Angle (deg)"; acamber "Camber Angle (deg)"; rod_mass "Mass (kg)"; whl_init_spd_lr "Initial Wheel Speed (rad/s)"; whlind "Wheel Index"
      mask help: This models a double-wishbone suspension for steered and non-steered configurations. The non-steered configuration maintains its orientation via the track rods that connect to fixed points on the subframe.
      mask init:
      | % sm_car_4post_lib_setLeftRight(gcb,'none');
      | 
      | if(popup_leftRight == 1)
      |     rhs_susp = 1;
      |     whlind = 1;
      | elseif(popup_leftRight == 2)
      |     rhs_susp = -1;
      |     whlind = 2;
      | end
      mask TypeOptions popup_leftRight: Left | Right
      mask TypeOptions hp_in_f_ua: Upper Arm/hp_in_f | Hardpoints/hp_in_f_ua
      mask TypeOptions hp_in_r_ua: Upper Arm/hp_in_r | Hardpoints/hp_in_r_ua
      mask TypeOptions hp_out_ua: Upper Arm/hp_out | Upright/hp_ua_out
      mask TypeOptions hp_in_f_la: Lower Arm/hp_in_f | Hardpoints/hp_in_f_la
      mask TypeOptions hp_in_r_la: Lower Arm/hp_in_r | Hardpoints/hp_in_r_la
      mask TypeOptions hp_out_la: Lower Arm/hp_out | Upright/hp_la_out
      mask TypeOptions hp_upr_cg: Upright/hp_upr_cg
      mask TypeOptions hp_upr_wc: Upright/hp_upr_wc
      mask TypeOptions hp_in_rod: Track Rod/hp_in
      mask TypeOptions hp_upr_rod: Track Rod/hp_out | Upright/hp_upr_rod
      mask TypeOptions hp_spr_top: Hardpoints/hp_spr_top | Shock/hp_spr_top
      mask TypeOptions hp_spr_bot: Lower Arm/hp_spr | Shock/hp_spr_bot
      mask TypeOptions clr_hp: Hardpoints/clr_hp
      mask TypeOptions opc_hp: Hardpoints/opc_hp
      mask TypeOptions size_hp: Hardpoints/size_hp
      mask TypeOptions ua_mass: Upper Arm/ua_mass
      mask TypeOptions clr_ua: Upper Arm/clr_ua
      mask TypeOptions opc_ua: Upper Arm/opc_ua
      mask TypeOptions radius_ua: Upper Arm/radius_ua
      mask TypeOptions la_mass: Lower Arm/la_mass
      mask TypeOptions clr_la: Lower Arm/clr_la
      mask TypeOptions opc_la: Lower Arm/opc_la
      mask TypeOptions radius_la: Lower Arm/radius_la
      mask TypeOptions shock_pist_mass: Shock/shock_pist_mass
      mask TypeOptions shock_cyl_mass: Shock/shock_cyl_mass
      mask TypeOptions up_lim_bumpstop: Shock/up_lim_bumpstop
      mask TypeOptions low_lim_bumpstop: Shock/low_lim_bumpstop
      mask TypeOptions clr_conn_shock: Shock/clr_conn_shock
      mask TypeOptions opc_conn_shock: Shock/opc_conn_shock
      mask TypeOptions size_conn_shock: Shock/size_conn_shock
      mask TypeOptions clr_shock_cyl: Shock/clr_shock_cyl
      mask TypeOptions opc_shock_cyl: Shock/opc_shock_cyl
      mask TypeOptions radius_shock_cyl: Shock/radius_shock_cyl
      mask TypeOptions clr_shock_piston: Shock/clr_shock_piston
      mask TypeOptions opc_shock_piston: Shock/opc_shock_piston
      mask TypeOptions clr_shock_bumpstop: Shock/clr_shock_bumpstop
      mask TypeOptions opc_shock_bumpstop: Shock/opc_shock_bumpstop
      mask TypeOptions deadvol_len_shock_cyl: Shock/deadvol_len_shock_cyl
      mask TypeOptions piston_len_shock: Shock/piston_len_shock
      mask TypeOptions cyl_cap_len_shock: Shock/cyl_cap_len_shock
      mask TypeOptions bumpstop_len_shock: Shock/bumpstop_len_shock
      mask TypeOptions upr_mass: Upright/upr_mass
      mask TypeOptions atoe: Upright/atoe
      mask TypeOptions acamber: Upright/acamber
      mask TypeOptions clr_conn_upr: Upright/clr_conn_upr
      mask TypeOptions opc_conn_upr: Upright/opc_conn_upr
      mask TypeOptions size_conn_upr: Upright/size_conn_upr
      mask TypeOptions clr_upr: Upright/clr_upr
      mask TypeOptions opc_upr: Upright/opc_upr
      mask TypeOptions radius_upr: Upright/radius_upr
      mask TypeOptions clr_stub_axle: Upright/clr_stub_axle
      mask TypeOptions opc_stub_axle: Upright/opc_stub_axle
      mask TypeOptions radius_stub_axle: Upright/radius_stub_axle
      mask TypeOptions rod_mass: Track Rod/rod_mass
      mask TypeOptions clr_conn_rod: Track Rod/clr_conn_rod
      mask TypeOptions opc_conn_rod: Track Rod/opc_conn_rod
      mask TypeOptions size_conn_rod: Track Rod/size_conn_rod
      mask TypeOptions clr_rod: Track Rod/clr_rod
      mask TypeOptions opc_rod: Track Rod/opc_rod
      mask TypeOptions radius_rod: Track Rod/radius_rod
      mask DialogControl cont_hp Prompt: Hardpoints
      mask DialogControl cont_vis_hp Prompt: Visualization
      mask DialogControl text_clr_hp Prompt: Color [RGB]
      mask DialogControl text_opc_hp Prompt: Opac. (0-1)
      mask DialogControl text_size_hp Prompt: Size (m)
      mask DialogControl text_hp Prompt: Hardpoints
      mask DialogControl cont_ua Prompt: UA
      mask DialogControl cont_vis_ua Prompt: Visualization
      mask DialogControl cont_la Prompt: LA
      mask DialogControl cont_vis_la Prompt: Visualization
      mask DialogControl cont_shock Prompt: Shock
      mask DialogControl cont_parts Prompt: Parts
      mask DialogControl cont_bumpstop Prompt: Bumpstop
      mask DialogControl cont_vis_shock Prompt: Visualization
      mask DialogControl text_clr_shock Prompt: Color  [RGB]
      mask DialogControl text_opc_shock Prompt: Opac. (0-1)
      mask DialogControl text_size_shock Prompt: Size (m)
      mask DialogControl text_conn_shock Prompt: Connections
      mask DialogControl text_shock_shock Prompt: Cylinder
      mask DialogControl text_shock_piston Prompt: Piston
      mask DialogControl text_piston_radius Prompt: <cylinder radius>
      mask DialogControl text_shock_bumpstop Prompt: Bumpstop
      mask DialogControl text_bumpstop_radius Prompt: <cylinder radius>
      mask DialogControl cont_upright Prompt: Upright
      mask DialogControl grp_upright Prompt: Upright
      mask DialogControl cont_vis_upr Prompt: Visualization
      mask DialogControl text_clr_upr Prompt: Color [RGB]
      mask DialogControl text_opc_upr Prompt: Opac. (0-1)
      mask DialogControl text_size_upr Prompt: Size (m)
      mask DialogControl text_conn_upr Prompt: Connections
      mask DialogControl text_upright Prompt: Upright
      mask DialogControl text_stub_axle Prompt: Stub Axle
      mask DialogControl cont_steer Prompt: Steer
      mask DialogControl grp_rod Prompt: Rod
      mask DialogControl cont_vis_rod Prompt: Visualization
      mask DialogControl text_clr_rod Prompt: Color [RGB]
      mask DialogControl text_opc_rod Prompt: Opac. (0-1)
      mask DialogControl text_size_rod Prompt: Size (m)
      mask DialogControl text_conn_rod Prompt: Connections
      mask DialogControl text_rod_rod Prompt: Rod
      mask DialogControl cont_init Prompt: Initial
  Rack : PMIOPort  Side=Right
  Ref : PMIOPort  Port=2  Side=Right
  Axle : PMIOPort  Port=3  Side=Left
  S : PMIOPort  Port=4  Side=Left
  D : PMIOPort  Port=5  Side=Left
  LAo : PMIOPort  Port=6  Side=Left
  WhlAng : Outport

== system MultibodySuspensionSSC/SuspR/Linkage/Anti Roll Bar ==
  " None" : Subsystem  VariantControl=None  mask(Anti-Roll Bar Placeholder){}
      mask help: Empty subsystem, used as a variant that omits an anti-roll bar.
  Simple : Subsystem  VariantControl=Simple  mask(Anti-Roll Bar, Simple){k=AntiRollBar.k.Value}
      mask prompts: k "Stiffness"
      mask help: Models an anti-roll bar by applying un-opposed forces to suspension arms. Conceptual use only.
  LAoL : PMIOPort  Side=Left
  Ref : PMIOPort  Port=2  Side=Left
  LAoR : PMIOPort  Port=3  Side=Left
